simulink model "DCMotor1FLC"  (R2018a)
settings: Solver=VariableStepAuto  StartTime=0.0  StopTime=6  MaxStep=0.01  RelTol=1e-4  EnableMultiTasking=on
undefined symbols (not defined in the file or in its folder): sigbuilder_block
libraries: fuzblock x1
settings Model: Creator=Nikos  LastModifiedBy=Panasavv
settings DataIOCC: LimitDataPoints=on  SaveOutput=off  SaveTime=off
settings OptimizationCC: ExpressionDepthLimit=2147483647  LifeSpan=1
settings DebuggingCC: UnderspecifiedInitializationDetection=Classic  MergeDetectMultiDrivingBlocksExec=none  FcnCallInpInsideContextMsg=warning  AllowSymbolicDim=off  StateNameClashWarn=warning  SFUnexpectedBacktrackingDiag=warning  SFNoUnconditionalDefaultTransitionDiag=warning  SFExecutionAtInitializationDiag=none
settings CodeAppCC: StateflowObjectComments=on
settings GRTTargetCC: TargetLangStandard=C89/C90 (ANSI)  GeneratePreprocessorConditionals=Disable all  CombineOutputUpdateFcns=off  GRTInterface=on

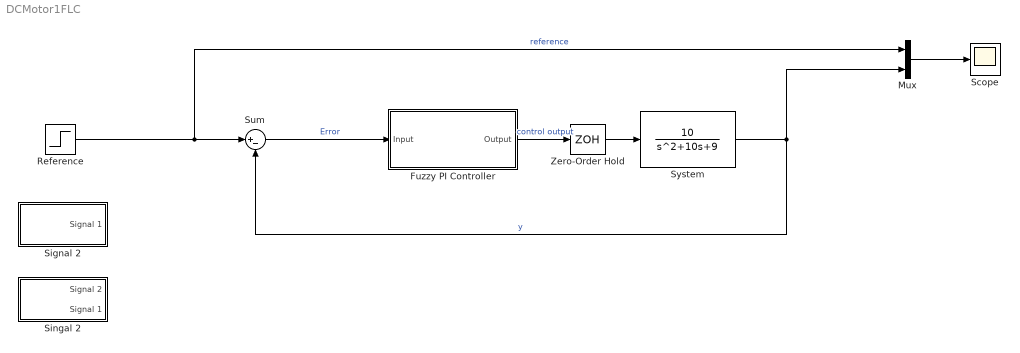
== system DCMotor1FLC ==
  "\tFuzzy PI Controller" : Subsystem
  Mux : Mux  Inputs=2
  Reference : Step  Time=0  SampleTime=0.01
  Scope : Scope
  Signal 2 : Subsystem  Tag=STV Subsys  LoadFcn=sigbuilder_block('load');  StartFcn=sigbuilder_block('start');  StopFcn=sigbuilder_block('stop');  ClipboardFcn=sigbuilder_block('clipboard');  mask(Sigbuilder block){tuvar=[0:10]}
      mask help: Simulink:masks:SigbuilderBlock_MD
      mask init:
      | if ~strcmp(get_param(bdroot(gcbh),'SimulationStatus'),'stopped') tuvar = sigbuilder_block('maskInit'); end
      settings: CopyFcn=sigbuilder_block('copy');  DeleteFcn=sigbuilder_block('delete');  ModelCloseFcn=sigbuilder_block('modelClose');  PreSaveFcn=sigbuilder_block('preSave');  PauseFcn=sigbuilder_block('pause');  ContinueFcn=sigbuilder_block('continue');  NameChangeFcn=sigbuilder_block('namechange');  OpenFcn=sigbuilder_block('open',[1440 0 1440 752.25 ]);  CloseFcn=sigbuilder_block('close');
      mask Display: plot(0, 0, 100, 100,[2, 2, 32, 32, 2], [68, 8, 8, 68, 68],[32, 2], [38, 38], [32, 19, 2],[53, 60, 44], [32, 17, 17, 2],[16, 16, 31, 31]);txt = getActiveGroup(gcbh);text(2, 100, txt,'verticalAlignment', 'top');
  Singal 2 : Subsystem  Tag=STV Subsys  LoadFcn=sigbuilder_block('load');  StartFcn=sigbuilder_block('start');  StopFcn=sigbuilder_block('stop');  ClipboardFcn=sigbuilder_block('clipboard');  mask(Sigbuilder block){tuvar=[0:10]}
      mask help: Simulink:masks:SigbuilderBlock_MD
      mask init:
      | if ~strcmp(get_param(bdroot(gcbh),'SimulationStatus'),'stopped') tuvar = sigbuilder_block('maskInit'); end
      settings: CopyFcn=sigbuilder_block('copy');  DeleteFcn=sigbuilder_block('delete');  ModelCloseFcn=sigbuilder_block('modelClose');  PreSaveFcn=sigbuilder_block('preSave');  PauseFcn=sigbuilder_block('pause');  ContinueFcn=sigbuilder_block('continue');  NameChangeFcn=sigbuilder_block('namechange');  OpenFcn=sigbuilder_block('open',[6 30 1428 681.75 ]);  CloseFcn=sigbuilder_block('close');
      mask Display: plot(0, 0, 100, 100,[2, 2, 32, 32, 2], [68, 8, 8, 68, 68],[32, 2], [38, 38], [32, 19, 2],[53, 60, 44], [32, 17, 17, 2],[16, 16, 31, 31]);txt = getActiveGroup(gcbh);text(2, 100, txt,'verticalAlignment', 'top');
  Sum : Sum  Inputs=|+-
  System : TransferFcn  Numerator=[10]  Denominator=[1 10 9]
  Zero-Order Hold : ZeroOrderHold  SampleTime=-1
  wires:
  "\tFuzzy PI Controller"/1(Output) -> Zero-Order Hold/1  "control output"
  Sum/1 -> "\tFuzzy PI Controller"/1(Input)  "Error"
  System/1 -> Mux/2, Sum/2  "y"
  Mux/1 -> Scope/1
  Zero-Order Hold/1 -> System/1
  Reference/1 -> Mux/1, Sum/1  "reference"

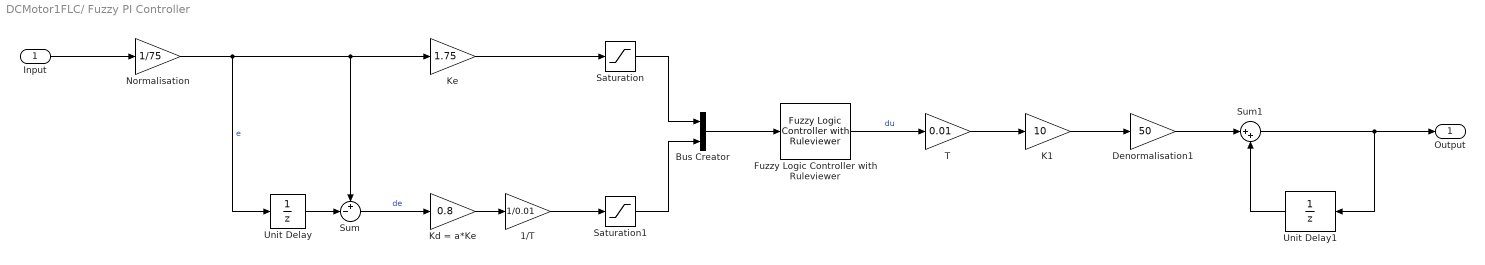
== system DCMotor1FLC/	Fuzzy PI Controller ==
  Input : Inport
  1/T : Gain  Gain=1/0.01
  Bus Creator : BusCreator  Inputs=2
  Denormalisation1 : Gain  Gain=50
  Fuzzy Logic Controller with Ruleviewer : fuzblock/Fuzzy Logic  Controller  with Ruleviewer  fismatrix=DCMotor1_Simulation  Ts=0.01
  K1 : Gain  Gain=10
  Kd = a*Ke : Gain  Gain=0.8
  Ke : Gain  Gain=1.75
  Normalisation : Gain  Gain=1/75
  Saturation : Saturate  UpperLimit=1  LowerLimit=-1
  Saturation1 : Saturate  UpperLimit=1  LowerLimit=-1
  Sum : Sum  Inputs=+-|
  Sum1 : Sum  Inputs=|++
  T : Gain  Gain=0.01
  Unit Delay : UnitDelay  SampleTime=-1
  Unit Delay1 : UnitDelay  SampleTime=-1
  Output : Outport
  wires:
  Input/1 -> Normalisation/1
  Normalisation/1 -> Ke/1, Sum/1, Unit Delay/1  "e"
  Unit Delay/1 -> Sum/2
  Sum/1 -> Kd = a*Ke/1  "de"
  Kd = a*Ke/1 -> 1/T/1
  1/T/1 -> Saturation1/1
  Ke/1 -> Saturation/1
  Bus Creator/1 -> Fuzzy Logic Controller with Ruleviewer/1
  Saturation/1 -> Bus Creator/1
  Saturation1/1 -> Bus Creator/2
  Fuzzy Logic Controller with Ruleviewer/1 -> T/1  "du"
  T/1 -> K1/1
  K1/1 -> Denormalisation1/1
  Denormalisation1/1 -> Sum1/1
  Sum1/1 -> Unit Delay1/1, Output/1
  Unit Delay1/1 -> Sum1/2

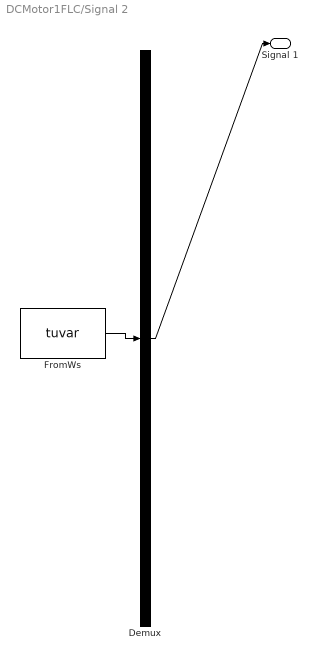
== system DCMotor1FLC/Signal 2 ==
  Demux : Demux  Tag=STV Demux  Outputs=1
  FromWs : FromWorkspace  Tag=STV FromWs  VariableName=tuvar  SampleTime=0
      SigBuilderData=|
      | common.afterFinalStr = 'Extrapolate'
      | common.sampleTime = 0
      | dataSet.timeRange = [0 35]
      | dataSet.name = 'Group 1'
      | sbobj.Groups.Name = 'Group 1'
      | sbobj.Groups.Signals.Name = 'Signal 1'
      | sbobj.Groups.Signals.XData = [0 10.02 20.04 20.04 30 35]
      | sbobj.Groups.Signals.YData = [0 150 150 149.5 0 0]
      | sbobj.Groups.TimeRange = [0 35]
  Signal 1 : Outport  Tag=STV Outport
  wires:
  FromWs/1 -> Demux/1
  Demux/1 -> Signal 1/1

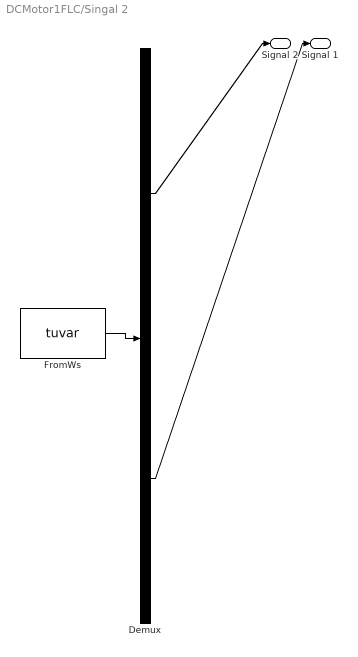
== system DCMotor1FLC/Singal 2 ==
  Demux : Demux  Tag=STV Demux  Outputs=2
  FromWs : FromWorkspace  Tag=STV FromWs  VariableName=tuvar  SampleTime=0
      SigBuilderData=|
      | common.afterFinalStr = 'Extrapolate'
      | common.sampleTime = 0
      | dataSet.timeRange = [0 30]
      | dataSet.name = 'Group 1'
      | sbobj.Groups.Name = 'Group 1'
      | sbobj.Groups.Signals(1).Name = 'Signal 2'
      | sbobj.Groups.Signals(1).XData = [0 30]
      | sbobj.Groups.Signals(1).YData = [150 150]
      | sbobj.Groups.Signals(2).Name = 'Signal 1'
      | sbobj.Groups.Signals(2).XData = [0 9.98 9.98 20.02 20.02 30]
      | sbobj.Groups.Signals(2).YData = [0 0 100 100 0 0]
      | sbobj.Groups.TimeRange = [0 30]
  Signal 2 : Outport  Tag=STV Outport
  Signal 1 : Outport  Tag=STV Outport  Port=2
  wires:
  FromWs/1 -> Demux/1
  Demux/1 -> Signal 2/1
  Demux/2 -> Signal 1/1
